simulink model "PubIfDecisionTOS_MDL"  (R2020b)
settings: configuration reference "DspaceConfig" (kept outside this file)
PostLoadFcn:
  | if any(exist('dsrtsu_mdlpostloadfcn', 'file') ~= 0), dsrtsu_mdlpostloadfcn('Execute', bdroot); end
InitFcn:
  | , if any(exist('dsmpb_private', 'file') ~= 0), dsmpb_private('dsmpb_mdlclblib', 'Init', bdroot); end,
undefined symbols (not defined in the file or in its folder): C_TOS_ACCEgoRAxletoFbumplength_m, C_TOS_ACCTargetFront_Flag, C_TOS_AEBJAPedObjDxThre_Val, C_TOS_AEBJAPedObjDyThre_Val, C_TOS_AEBJATargetSize_Val, C_TOS_AEBJAVehObjDxThre_Val, C_TOS_AEBJAVehObjDyThre_Val, C_TOS_AEBJuncPedTargetSize_Val, C_TOS_AEBLatObjDxThre_Val, C_TOS_AEBLatPedDyThre_Val, C_TOS_AEBLatTargetSize_Val, C_TOS_AEBLongTargetInEgoFront_Flag, C_TOS_axAbsGround_Parameter, C_TOS_CameraConfirmedFlag, C_TOS_CNsubjWidth, C_TOS_CurrentLaneCoreMinWidth_Val, C_TOS_CutInProb_Val_Zero, C_TOS_CutOutProb_Val_Zero, C_TOS_D2R_Val, C_TOS_DefaultValueObjectToCenterLine_dy, C_TOS_EgoCarWidth_Val, C_TOS_EgoDxRefPoint_m, C_TOS_EgoRAxletoFbumplength_m, C_TOS_HalfWidthVehicle_Con, C_TOS_HWA_CurrentLaneFlag, C_TOS_HWA_LeftLaneFlag, C_TOS_HWA_MovingDir_Vaild, C_TOS_HWA_MovState_Vaild, C_TOS_HWA_RightLaneFlag, C_TOS_LaneLineCourseErrorFront, C_TOS_LaneLineCourseErrorRear, C_TOS_MotorbikeDefaultWidth_m, C_TOS_NumberOfEffectiveTargets, C_TOS_Obj_Age_Val, C_TOS_Objdx_Constraint_Val, C_TOS_ObjectDefaultWidth_m, C_TOS_ObjInCurrentLane_Val, C_TOS_ObjInCurrentLaneValid, C_TOS_ObjInLeftLaneValid, C_TOS_ObjInRightLaneValid, C_TOS_ObjNotInCurrentLane_Val, C_TOS_ObjNotREElementType, C_TOS_ObjPredictDis_dy_ConstantVal_Zeros, C_TOS_ObjToCenterLine_ConstantVal_Zeros, C_TOS_OFMObjIDInvilad_Val, C_TOS_PIL_LatDisCons_Val_zero, C_TOS_PIL_ObjectCutInFlag_b, C_TOS_PIL_ObjectCutOutFlag_b, C_TOS_PIL_ObjLaneProb_al_Val, C_TOS_PP_ObjFusType_FC_Confirm_b, C_TOS_PP_ObjFusType_FC_FR_Confirm_b, C_TOS_PP_ObjFusType_FR_Confirm_b, C_TOS_RE_80BoolDefault_Val, C_TOS_RE_80Single181Default_Val, C_TOS_RE_80Single255Default_Val, C_TOS_RE_80Uint8Default_Val, C_TOS_RE_D2R, C_TOS_RE_D_180_Val, C_TOS_RE_InvalidObjectID_Val, C_TOS_RE_InvalidTargetChainDir_Val ... (+142)
libraries: simulink x1650, TOS_LIB x361, canfdmsglib x14
(part 56 of 69)

== system PubIfDecisionTOS_MDL/TOS_20201112/TOS_2012080320/TOS/LC_LCKie_ELK/TOS_HWA/LeftLane/TOS_HWA_LeftLane/TOS_HWA_LeftLane/TOS_HWA/HWA_LeftLane/HWA_LeftLane_Rear ==
  HWA_MovState_InternalSig : Inport
  Object_Fus_Type : Inport  Port=2
  TOS_TLJ_LeftLaneConfirm_Flag : Inport  Port=3
  HWA_MovingDir_InternalSig : Inport  Port=4
  Object_DY : Inport  Port=5
  Object_DX : Inport  Port=6
  HWA_InLeftLane_Flag : Subsystem
  HWA_LeftFront_Default : Subsystem
  HWA_LeftRear_DyConfirm : Subsystem
  HWA_LeftRear_FusionType : Subsystem
  HWA_LeftRear_MovState : Subsystem
  HWA_LeftRear_TargetMovingDir : Subsystem
  Logical Operator4 : Logic  Inputs=5  AllPortsSameDT=off  OutDataTypeStr=boolean
  Object_DX1 : InportShadow  Port=6
  TOS_HWA_LeftFront_TargConfirm_b : Outport
  TOS_HWA_LeftFront_FusType_ObserVale : Outport  Port=2
  TOS_HWA_InLeftLane_Front_Flag_ObserVale : Outport  Port=3
  TOS_HWA_LeftFront_TargMovDir_ObserVale : Outport  Port=4
  TOS_HWA_LeftRear_TargConfirm_b : Outport  Port=5
  TOS_HWA_LeftRear_MovState_ObserVale : Outport  Port=6
  TOS_HWA_LeftRear_FusionType_ObserVale : Outport  Port=7
  TOS_HWA_InLeftLane_Rear_Flag_ObserVale : Outport  Port=8
  TOS_HWA_LeftRear_TargetMovingDir_ObserVale : Outport  Port=9
  TOS_HWA_LeftRear_DyConfirm_ObserVale : Outport  Port=10
  wires:
  Object_DX1/1 -> HWA_LeftRear_FusionType/2(Object_DX)
  Object_DX/1 -> HWA_LeftRear_DyConfirm/2(Object_DX)
  HWA_LeftRear_DyConfirm/1(TOS_HWA_LeftRear_DyConfirm) -> Logical Operator4/5, [TOS_HWA_LeftRear_DyConfirm_ObserVale]
  HWA_LeftRear_TargetMovingDir/1(TOS_HWA_LeftRear_TargetMovingDir) -> Logical Operator4/4, [TOS_HWA_LeftRear_TargetMovingDir_ObserVale]
  HWA_InLeftLane_Flag/1(TOS_HWA_InLeftLane_Flag) -> Logical Operator4/3, [TOS_HWA_InLeftLane_Flag_ObserVale]
  HWA_LeftRear_FusionType/1(TOS_HWA_LeftRear_FusionType) -> Logical Operator4/2, [TOS_HWA_LeftRear_FusionType_ObserVale]
  HWA_LeftRear_MovState/1(TOS_HWA_LeftRear_MovState) -> Logical Operator4/1, [TOS_HWA_LeftRear_MovState_ObserVale]
  Object_DY/1 -> HWA_LeftRear_DyConfirm/1(Object_DY)
  HWA_MovingDir_InternalSig/1 -> HWA_LeftRear_TargetMovingDir/1(HWA_MovingDir_InternalSig)
  TOS_TLJ_LeftLaneConfirm_Flag/1 -> HWA_InLeftLane_Flag/1(HWA_InRightLane)
  Object_Fus_Type/1 -> HWA_LeftRear_FusionType/1(Object_FusType)
  HWA_MovState_InternalSig/1 -> HWA_LeftRear_MovState/1(HWA_MovState_InternalSig)
  [TOS_HWA_LeftRear_DyConfirm_ObserVale] -> TOS_HWA_LeftRear_DyConfirm_ObserVale/1  "TOS_HWA_LeftRear_DyConfirm_ObserVale"
  [TOS_HWA_LeftRear_TargetMovingDir_ObserVale] -> TOS_HWA_LeftRear_TargetMovingDir_ObserVale/1  "TOS_HWA_LeftRear_TargetMovingDir_ObserVale"
  Logical Operator4/1 -> TOS_HWA_LeftRear_TargConfirm_b/1  "TOS_HWA_LeftRear_TargConfirm_b"
  HWA_LeftFront_Default/3(TOS_HWA_InLeftLane_Front_Flag_ObserVale) -> TOS_HWA_InLeftLane_Front_Flag_ObserVale/1  "TOS_HWA_InLeftLane_Front_Flag_ObserVale"
  HWA_LeftFront_Default/2(TOS_HWA_LeftFront_FusType_ObserVale) -> TOS_HWA_LeftFront_FusType_ObserVale/1  "TOS_HWA_LeftFront_FusType_ObserVale"
  [TOS_HWA_InLeftLane_Flag_ObserVale] -> TOS_HWA_InLeftLane_Rear_Flag_ObserVale/1  "TOS_HWA_InLeftLane_Rear_Flag_ObserVale"
  HWA_LeftFront_Default/1(TOS_HWA_LeftFront_TargConfirm_b) -> TOS_HWA_LeftFront_TargConfirm_b/1  "TOS_HWA_LeftFront_TargConfirm_b"
  HWA_LeftFront_Default/4(TOS_HWA_LeftFront_TargMovDir_ObserVale) -> TOS_HWA_LeftFront_TargMovDir_ObserVale/1  "TOS_HWA_LeftFront_TargMovDir_ObserVale"
  [TOS_HWA_LeftRear_MovState_ObserVale] -> TOS_HWA_LeftRear_MovState_ObserVale/1  "TOS_HWA_LeftRear_MovState_ObserVale"
  [TOS_HWA_LeftRear_FusionType_ObserVale] -> TOS_HWA_LeftRear_FusionType_ObserVale/1  "TOS_HWA_LeftRear_FusionType_ObserVale"

== system PubIfDecisionTOS_MDL/TOS_20201112/TOS_2012080320/TOS/LC_LCKie_ELK/TOS_HWA/LeftLane/TOS_HWA_LeftLane/TOS_HWA_LeftLane/TOS_HWA/HWA_LeftLane/HWA_MovState ==
  note: Fun：计算目标相对于大地的绝对速度
      |
      | fun1:目标绝对速度 = 目标相对速度（融合输出）+ 自车速度
      |
      | （目标相对速度 = 目标速度 - 自车速度）
  Object_VX : Inport
  Object_VY : Inport  Port=2
  VIE_EgoVelocity : Inport  Port=3
  Add : Sum
  Compare To Constant1 : simulink/Logic and Bit Operations/Compare To Constant  relop=>  const=1.5  OutDataTypeStr=boolean
      settings: AttributesFormatString== 1.5
  Terminator : Terminator
  HWA_MovState_InternalSig : Outport
  wires:
  Compare To Constant1/1 -> HWA_MovState_InternalSig/1
  Object_VY/1 -> Terminator/1
  Add/1 -> Compare To Constant1/1
  VIE_EgoVelocity/1 -> Add/2
  Object_VX/1 -> Add/1

== system PubIfDecisionTOS_MDL/TOS_20201112/TOS_2012080320/TOS/LC_LCKie_ELK/TOS_HWA/LeftLane/TOS_HWA_LeftLane/TOS_HWA_LeftLane/TOS_HWA/HWA_LeftLane/HWA_MovingDir ==
  note: OncomingDir
  note: SameDir
  object_MovingState : Inport
  PP_ObjMovingDirSignalProcessing : Inport  Port=2
  Object_HeadingAngle : Inport  Port=3
  Object_VX : Inport  Port=4
  Object_VY : Inport  Port=5
  VIE_EgoVelocity : Inport  Port=6
  Abs{,1..3} (4 alike) : Abs
  Add : Sum
  Add1 : Sum
  Compare To Constant : simulink/Logic and Bit Operations/Compare To Constant  relop===  const=ObjectMovingOrientation_E.SameDir  OutDataTypeStr=boolean
      settings: AttributesFormatString=ObjectMovingOrientation_E.SameDir = 1
  Compare To Constant1 : simulink/Logic and Bit Operations/Compare To Constant  relop===  const=OFM_OBJ_MOVINGSTATE_E.MOVING  OutDataTypeStr=boolean
      settings: AttributesFormatString=OFM_OBJ_MOVINGSTATE_E.MOVING = 2
  Compare To Constant2 : simulink/Logic and Bit Operations/Compare To Constant  relop=>=  const=P_TOS_ObjInSameDirYawAngMinThre_Val  OutDataTypeStr=boolean
      settings: AttributesFormatString=P_TOS_ObjInSameDirYawAngMinThre_Val = 0
  Compare To Constant3 : simulink/Logic and Bit Operations/Compare To Constant  relop=<=  const=P_TOS_ObjInSameDirYawAngMaxThre_Val  OutDataTypeStr=boolean
      settings: AttributesFormatString=P_TOS_ObjInSameDirYawAngMaxThre_Val = 45
  Compare To Constant4 : simulink/Logic and Bit Operations/Compare To Constant  relop===  const=OFM_OBJ_MOVINGSTATE_E.MOVING_SLOWLY  OutDataTypeStr=boolean
      settings: AttributesFormatString=OFM_OBJ_MOVINGSTATE_E.MOVING_SLOWLY = 5
  Compare To Constant5 : simulink/Logic and Bit Operations/Compare To Constant  relop===  const=ObjectMovingOrientation_E.OnComingDir  OutDataTypeStr=boolean
      settings: AttributesFormatString=ObjectMovingOrientation_E.OnComingDir = 2
  Compare To Constant6 : simulink/Logic and Bit Operations/Compare To Constant  relop=>=  const=P_TOS_ObjLatCroYawAngMaxThre_Val  OutDataTypeStr=boolean
      settings: AttributesFormatString=P_TOS_ObjLatCroYawAngMaxThre_Val = 135
  Compare To Constant7 : simulink/Logic and Bit Operations/Compare To Constant  relop=<=  const=P_TOS_ObjOncomingYawAngMaxThre_Val  OutDataTypeStr=boolean
      settings: AttributesFormatString=P_TOS_ObjOncomingYawAngMaxThre_Val = 180
  Compare To Constant8 : simulink/Logic and Bit Operations/Compare To Constant  relop=<  const=P_TOS_SameDirVyOffset_Val  OutDataTypeStr=boolean
      settings: AttributesFormatString=P_TOS_SameDirVyOffset_Val = 2
  Constant : Constant  OutDataTypeStr=boolean
  Constant1 : Constant  Value=P_TOS_SameDirVxvOffset_Val
      settings: AttributesFormatString=P_TOS_AEBLong_SameDirVxvOffset_Val = 0.2
  Constant2 : Constant  Value=P_TOS_OncomingDirVxvOffset_Val
      settings: AttributesFormatString=P_TOS_OncomingDirVxvOffset_Val = 0.2
  Data Type Conversion1 : DataTypeConversion  OutDataTypeStr=Enum: ObjectMovingOrientation_E
  Data Type Conversion2 : DataTypeConversion  OutDataTypeStr=Enum: OFM_OBJ_MOVINGSTATE_E
  Logical Operator{,3..4,7} (4 alike) : Logic  AllPortsSameDT=off  OutDataTypeStr=boolean
  Logical Operator1 : Logic  Operator=OR  AllPortsSameDT=off  OutDataTypeStr=boolean
  Logical Operator2 : Logic  Operator=OR  AllPortsSameDT=off  OutDataTypeStr=boolean
  Logical Operator5 : Logic  Operator=OR  AllPortsSameDT=off  OutDataTypeStr=boolean
  Logical Operator6 : Logic  Operator=OR  Inputs=4  AllPortsSameDT=off  OutDataTypeStr=boolean
  Relational Operator : RelationalOperator  Operator=<  OutDataTypeStr=boolean  RndMeth=Simplest
  Relational Operator1 : RelationalOperator  Operator=>  OutDataTypeStr=boolean  RndMeth=Simplest
  Switch : Switch  Criteria=u2 > Threshold
  HWA_MovingDir_InternalSig : Outport
  wires:
  Abs3/1 -> Add1/1
  [VIE_EgoVelocity] -> Relational Operator1/2
  Add1/1 -> Relational Operator1/1
  Logical Operator7/1 -> Logical Operator6/4
  Relational Operator1/1 -> Logical Operator7/2
  Logical Operator/1 -> Logical Operator6/3
  [Object_VX] -> Abs3/1
  Abs2/1 -> Compare To Constant8/1
  Object_VY/1 -> Abs2/1
  Add/1 -> Relational Operator/1
  Constant1/1 -> Add/2
  Object_VX/1 -> Abs1/1, [Object_VX]
  VIE_EgoVelocity/1 -> [VIE_EgoVelocity], Relational Operator/2
  Abs1/1 -> Add/1
  Compare To Constant8/1 -> Logical Operator/2, Logical Operator7/1
  Relational Operator/1 -> Logical Operator/1
  Constant2/1 -> Add1/2
  Logical Operator1/1 -> Logical Operator6/2
  Logical Operator5/1 -> Logical Operator6/1
  Compare To Constant5/1 -> Logical Operator5/1
  Logical Operator4/1 -> Logical Operator5/2
  Compare To Constant7/1 -> Logical Operator4/2
  Compare To Constant6/1 -> Logical Operator4/1
  PP_ObjMovingDirSignalProcessing/1 -> Data Type Conversion1/1
  Logical Operator6/1 -> Switch/1
  Data Type Conversion1/1 -> Compare To Constant5/1, Compare To Constant/1
  Compare To Constant2/1 -> Logical Operator3/1
  Compare To Constant3/1 -> Logical Operator3/2
  Abs/1 -> Compare To Constant6/1, Compare To Constant3/1, Compare To Constant2/1, Compare To Constant7/1
  Object_HeadingAngle/1 -> Abs/1
  Compare To Constant/1 -> Logical Operator1/1
  Logical Operator3/1 -> Logical Operator1/2
  Data Type Conversion2/1 -> Compare To Constant4/1, Compare To Constant1/1
  object_MovingState/1 -> Data Type Conversion2/1
  Compare To Constant4/1 -> Logical Operator2/2
  Compare To Constant1/1 -> Logical Operator2/1
  Logical Operator2/1 -> Switch/2
  Switch/1 -> HWA_MovingDir_InternalSig/1
  Constant/1 -> Switch/3

== system PubIfDecisionTOS_MDL/TOS_20201112/TOS_2012080320/TOS/LC_LCKie_ELK/TOS_HWA/RightLane/TOS_HWA_RightLane/TOS_HWA_RightLane/TOS_HWA/HWA_RightLane/HWA_MovState ==
  note: Fun：计算目标相对于大地的绝对速度
      |
      | fun1:目标绝对速度 = 目标相对速度（融合输出）+ 自车速度
      |
      | （目标相对速度 = 目标速度 - 自车速度）
  Object_VX : Inport
  Object_VY : Inport  Port=2
  VIE_EgoVelocity : Inport  Port=3
  Add : Sum
  Compare To Constant1 : simulink/Logic and Bit Operations/Compare To Constant  relop=>  const=1.5  OutDataTypeStr=boolean
      settings: AttributesFormatString== 1.5
  Terminator : Terminator
  HWA_MovState_InternalSig : Outport
  wires:
  Object_VX/1 -> Add/1
  VIE_EgoVelocity/1 -> Add/2
  Add/1 -> Compare To Constant1/1
  Object_VY/1 -> Terminator/1
  Compare To Constant1/1 -> HWA_MovState_InternalSig/1

== system PubIfDecisionTOS_MDL/TOS_20201112/TOS_2012080320/TOS/LC_LCKie_ELK/TOS_HWA/RightLane/TOS_HWA_RightLane/TOS_HWA_RightLane/TOS_HWA/HWA_RightLane/HWA_MovingDir ==
  note: SameDir
  note: OncomingDir
  object_MovingState : Inport
  PP_ObjMovingDirSignalProcessing : Inport  Port=2
  Object_HeadingAngle : Inport  Port=3
  Object_VX : Inport  Port=4
  Object_VY : Inport  Port=5
  VIE_EgoVelocity : Inport  Port=6
  Abs{,1..3} (4 alike) : Abs
  Add : Sum
  Add1 : Sum
  Compare To Constant : simulink/Logic and Bit Operations/Compare To Constant  relop===  const=ObjectMovingOrientation_E.SameDir  OutDataTypeStr=boolean
      settings: AttributesFormatString=ObjectMovingOrientation_E.SameDir = 1
  Compare To Constant1 : simulink/Logic and Bit Operations/Compare To Constant  relop===  const=OFM_OBJ_MOVINGSTATE_E.MOVING  OutDataTypeStr=boolean
      settings: AttributesFormatString=OFM_OBJ_MOVINGSTATE_E.MOVING = 2
  Compare To Constant2 : simulink/Logic and Bit Operations/Compare To Constant  relop=>=  const=P_TOS_ObjInSameDirYawAngMinThre_Val  OutDataTypeStr=boolean
      settings: AttributesFormatString=P_TOS_ObjInSameDirYawAngMinThre_Val = 0
  Compare To Constant3 : simulink/Logic and Bit Operations/Compare To Constant  relop=<=  const=P_TOS_ObjInSameDirYawAngMaxThre_Val  OutDataTypeStr=boolean
      settings: AttributesFormatString=P_TOS_ObjInSameDirYawAngMaxThre_Val = 45
  Compare To Constant4 : simulink/Logic and Bit Operations/Compare To Constant  relop===  const=OFM_OBJ_MOVINGSTATE_E.MOVING_SLOWLY  OutDataTypeStr=boolean
      settings: AttributesFormatString=OFM_OBJ_MOVINGSTATE_E.MOVING_SLOWLY = 5
  Compare To Constant5 : simulink/Logic and Bit Operations/Compare To Constant  relop===  const=ObjectMovingOrientation_E.OnComingDir  OutDataTypeStr=boolean
      settings: AttributesFormatString=ObjectMovingOrientation_E.OnComingDir = 2
  Compare To Constant6 : simulink/Logic and Bit Operations/Compare To Constant  relop=>=  const=P_TOS_ObjLatCroYawAngMaxThre_Val  OutDataTypeStr=boolean
      settings: AttributesFormatString=P_TOS_ObjLatCroYawAngMaxThre_Val = 135
  Compare To Constant7 : simulink/Logic and Bit Operations/Compare To Constant  relop=<=  const=P_TOS_ObjOncomingYawAngMaxThre_Val  OutDataTypeStr=boolean
      settings: AttributesFormatString=P_TOS_ObjOncomingYawAngMaxThre_Val = 180
  Compare To Constant8 : simulink/Logic and Bit Operations/Compare To Constant  relop=<  const=P_TOS_SameDirVyOffset_Val  OutDataTypeStr=boolean
      settings: AttributesFormatString=P_TOS_SameDirVyOffset_Val = 2
  Constant : Constant  OutDataTypeStr=boolean
  Constant1 : Constant  Value=P_TOS_SameDirVxvOffset_Val
      settings: AttributesFormatString=P_TOS_AEBLong_SameDirVxvOffset_Val = 0.2
  Constant2 : Constant  Value=P_TOS_OncomingDirVxvOffset_Val
      settings: AttributesFormatString=P_TOS_OncomingDirVxvOffset_Val = 0.2
  Data Type Conversion1 : DataTypeConversion  OutDataTypeStr=Enum: ObjectMovingOrientation_E
  Data Type Conversion2 : DataTypeConversion  OutDataTypeStr=Enum: OFM_OBJ_MOVINGSTATE_E
  Logical Operator{,3..4,7} (4 alike) : Logic  AllPortsSameDT=off  OutDataTypeStr=boolean
  Logical Operator1 : Logic  Operator=OR  AllPortsSameDT=off  OutDataTypeStr=boolean
  Logical Operator2 : Logic  Operator=OR  AllPortsSameDT=off  OutDataTypeStr=boolean
  Logical Operator5 : Logic  Operator=OR  AllPortsSameDT=off  OutDataTypeStr=boolean
  Logical Operator6 : Logic  Operator=OR  Inputs=4  AllPortsSameDT=off  OutDataTypeStr=boolean
  Relational Operator : RelationalOperator  Operator=<  OutDataTypeStr=boolean  RndMeth=Simplest
  Relational Operator1 : RelationalOperator  Operator=>  OutDataTypeStr=boolean  RndMeth=Simplest
  Switch : Switch  Criteria=u2 > Threshold
  HWA_MovingDir_InternalSig : Outport
  wires:
  Constant/1 -> Switch/3
  Switch/1 -> HWA_MovingDir_InternalSig/1
  Logical Operator2/1 -> Switch/2
  Compare To Constant1/1 -> Logical Operator2/1
  Compare To Constant4/1 -> Logical Operator2/2
  object_MovingState/1 -> Data Type Conversion2/1
  Data Type Conversion2/1 -> Compare To Constant1/1, Compare To Constant4/1
  Logical Operator3/1 -> Logical Operator1/2
  Compare To Constant/1 -> Logical Operator1/1
  Object_HeadingAngle/1 -> Abs/1
  Abs/1 -> Compare To Constant7/1, Compare To Constant2/1, Compare To Constant3/1, Compare To Constant6/1
  Compare To Constant3/1 -> Logical Operator3/2
  Compare To Constant2/1 -> Logical Operator3/1
  Data Type Conversion1/1 -> Compare To Constant/1, Compare To Constant5/1
  Logical Operator6/1 -> Switch/1
  PP_ObjMovingDirSignalProcessing/1 -> Data Type Conversion1/1
  Compare To Constant6/1 -> Logical Operator4/1
  Compare To Constant7/1 -> Logical Operator4/2
  Logical Operator4/1 -> Logical Operator5/2
  Compare To Constant5/1 -> Logical Operator5/1
  Logical Operator5/1 -> Logical Operator6/1
  Logical Operator1/1 -> Logical Operator6/2
  Constant2/1 -> Add1/2
  Relational Operator/1 -> Logical Operator/1
  Compare To Constant8/1 -> Logical Operator7/1, Logical Operator/2
  Abs1/1 -> Add/1
  VIE_EgoVelocity/1 -> Relational Operator/2, [VIE_EgoVelocity]
  Object_VX/1 -> [Object_VX], Abs1/1
  Constant1/1 -> Add/2
  Add/1 -> Relational Operator/1
  Object_VY/1 -> Abs2/1
  Abs2/1 -> Compare To Constant8/1
  [Object_VX] -> Abs3/1
  Logical Operator/1 -> Logical Operator6/3
  Relational Operator1/1 -> Logical Operator7/2
  Logical Operator7/1 -> Logical Operator6/4
  Add1/1 -> Relational Operator1/1
  [VIE_EgoVelocity] -> Relational Operator1/2
  Abs3/1 -> Add1/1

== system PubIfDecisionTOS_MDL/TOS_20201112/TOS_2012080320/TOS/LC_LCKie_ELK/TOS_HWA/RightLane/TOS_HWA_RightLane/TOS_HWA_RightLane/TOS_HWA/HWA_RightLane/HWA_RightLane_Default ==
  Constant{,1..9} (10 alike) : Constant  Value=0  OutDataTypeStr=boolean
  TOS_HWA_RightFront_TargConfirm_b : Outport
  TOS_HWA_RightFront_FusType_ObserVale : Outport  Port=2
  TOS_HWA_InRightLane_Front_Flag_ObserVale : Outport  Port=3
  TOS_HWA_RightFront_TargMovDir_ObserVale : Outport  Port=4
  TOS_HWA_RightRear_TargConfirm_b : Outport  Port=5
  TOS_HWA_RightRear_MovState_ObserVale : Outport  Port=6
  TOS_HWA_RightRear_FusionType_ObserVale : Outport  Port=7
  TOS_HWA_InRightLane_Rear_Flag_ObserVale : Outport  Port=8
  TOS_HWA_RightRear_TargetMovingDir_ObserVale : Outport  Port=9
  TOS_HWA_RightRear_DyConfirm_ObserVale : Outport  Port=10
  wires:
  Constant3/1 -> TOS_HWA_RightFront_TargMovDir_ObserVale/1  "TOS_HWA_RightFront_TargMovDir_ObserVale"
  Constant/1 -> TOS_HWA_RightFront_TargConfirm_b/1  "TOS_HWA_RightFront_TargConfirm_b"
  Constant1/1 -> TOS_HWA_RightFront_FusType_ObserVale/1  "TOS_HWA_RightFront_FusType_ObserVale"
  Constant6/1 -> TOS_HWA_RightRear_FusionType_ObserVale/1  "TOS_HWA_RightRear_FusionType_ObserVale"
  Constant7/1 -> TOS_HWA_InRightLane_Rear_Flag_ObserVale/1  "TOS_HWA_InRightLane_Rear_Flag_ObserVale"
  Constant9/1 -> TOS_HWA_RightRear_DyConfirm_ObserVale/1  "TOS_HWA_RightRear_DyConfirm_ObserVale"
  Constant8/1 -> TOS_HWA_RightRear_TargetMovingDir_ObserVale/1  "TOS_HWA_RightRear_TargetMovingDir_ObserVale"
  Constant5/1 -> TOS_HWA_RightRear_MovState_ObserVale/1  "TOS_HWA_RightRear_MovState_ObserVale"
  Constant2/1 -> TOS_HWA_InRightLane_Front_Flag_ObserVale/1  "TOS_HWA_InRightLane_Front_Flag_ObserVale"
  Constant4/1 -> TOS_HWA_RightRear_TargConfirm_b/1  "TOS_HWA_RightRear_TargConfirm_b"

== system PubIfDecisionTOS_MDL/TOS_20201112/TOS_2012080320/TOS/LC_LCKie_ELK/TOS_HWA/RightLane/TOS_HWA_RightLane/TOS_HWA_RightLane/TOS_HWA/HWA_RightLane/HWA_RightLane_Front ==
  object_MovingState : Inport
  PP_ObjFusType_FR_Confirm : Inport  Port=2
  PP_ObjFusType_FC_Confirm : Inport  Port=3
  HWA_MovState_InternalSig : Inport  Port=4
  TOS_TLJ_RightLaneConfirm_Flag : Inport  Port=5
  HWA_MovingDir_InternalSig : Inport  Port=6
  Object_DX : Inport  Port=7
  Bus Creator : BusCreator  Inputs=7
  Bus Selector : BusSelector  OutputSignals=object_MovingState,PP_ObjFusType_FR_Confirm,PP_ObjFusType_FC_Confirm,HWA_MovState_InternalSig,Object_DX
  Bus Selector1 : BusSelector  OutputSignals=TOS_TLJ_RightLaneConfirm_Flag
  Bus Selector2 : BusSelector  OutputSignals=HWA_MovingDir_InternalSig
  HWA_InRightLane_Flag : Subsystem
  HWA_RightFront_FusType : Subsystem
  HWA_RightFront_TargMovDir : Subsystem
  HWA_RightRear_Default : Subsystem
  Logical Operator4 : Logic  Inputs=3  AllPortsSameDT=off  OutDataTypeStr=boolean
  TOS_HWA_RightFront_TargConfirm_b : Outport
  TOS_HWA_RightFront_FusType_ObserVale : Outport  Port=2
  TOS_HWA_InRightLane_Front_Flag_ObserVale : Outport  Port=3
  TOS_HWA_RightFront_TargMovDir_ObserVale : Outport  Port=4
  TOS_HWA_RightRear_TargConfirm_b : Outport  Port=5
  TOS_HWA_RightRear_MovState_ObserVale : Outport  Port=6
  TOS_HWA_RightRear_FusionType_ObserVale : Outport  Port=7
  TOS_HWA_InRightLane_Rear_Flag_ObserVale : Outport  Port=8
  TOS_HWA_RightRear_TargetMovingDir_ObserVale : Outport  Port=9
  TOS_HWA_RightRear_DyConfirm_ObserVale : Outport  Port=10
  wires:
  object_MovingState/1 -> Bus Creator/1  "object_MovingState"
  HWA_MovingDir_InternalSig/1 -> Bus Creator/6  "HWA_MovingDir_InternalSig"
  TOS_TLJ_RightLaneConfirm_Flag/1 -> Bus Creator/5  "TOS_TLJ_RightLaneConfirm_Flag"
  HWA_MovState_InternalSig/1 -> Bus Creator/4  "HWA_MovState_InternalSig"
  PP_ObjFusType_FC_Confirm/1 -> Bus Creator/3  "PP_ObjFusType_FC_Confirm"
  PP_ObjFusType_FR_Confirm/1 -> Bus Creator/2  "PP_ObjFusType_FR_Confirm"
  Bus Creator/1 -> Bus Selector2/1, Bus Selector1/1, Bus Selector/1
  Bus Selector/1 -> HWA_RightFront_FusType/1(object_MovingState)  "<object_MovingState>"
  Bus Selector/2 -> HWA_RightFront_FusType/2(PP_ObjFusType_FR_Confirm)  "<PP_ObjFusType_FR_Confirm>"
  Bus Selector/3 -> HWA_RightFront_FusType/3(PP_ObjFusType_FC_Confirm)  "<PP_ObjFusType_FC_Confirm>"
  Bus Selector/4 -> HWA_RightFront_FusType/4(HWA_MovState_InternalSig)  "<HWA_MovState_InternalSig>"
  Bus Selector1/1 -> HWA_InRightLane_Flag/1(TOS_TLJ_RightLaneConfirm_Flag)  "<TOS_TLJ_RightLaneConfirm_Flag>"
  Bus Selector2/1 -> HWA_RightFront_TargMovDir/1(HWA_MovingDir_InternalSig)  "<HWA_MovingDir_InternalSig>"
  HWA_RightFront_FusType/1(TOS_HWA_RightFront_FusType) -> [TOS_HWA_RightFront_FusType_ObserVale], Logical Operator4/1
  HWA_InRightLane_Flag/1(TOS_HWA_InRightLane_Flag) -> [TOS_HWA_InRightLane_Flag_ObserVale], Logical Operator4/2
  HWA_RightFront_TargMovDir/1(TOS_HWA_RightFront_TargMovDir) -> [TOS_HWA_RightFront_TargMovDir_ObserVale], Logical Operator4/3
  Logical Operator4/1 -> TOS_HWA_RightFront_TargConfirm_b/1  "TOS_HWA_RightFront_TargConfirm_b"
  [TOS_HWA_RightFront_FusType_ObserVale] -> TOS_HWA_RightFront_FusType_ObserVale/1  "TOS_HWA_RightFront_FusType_ObserVale"
  [TOS_HWA_InRightLane_Flag_ObserVale] -> TOS_HWA_InRightLane_Front_Flag_ObserVale/1  "TOS_HWA_InRightLane_Front_Flag_ObserVale"
  [TOS_HWA_RightFront_TargMovDir_ObserVale] -> TOS_HWA_RightFront_TargMovDir_ObserVale/1  "TOS_HWA_RightFront_TargMovDir_ObserVale"
  HWA_RightRear_Default/1(TOS_HWA_RightRear_TargConfirm_b) -> TOS_HWA_RightRear_TargConfirm_b/1  "TOS_HWA_RightRear_TargConfirm_b"
  HWA_RightRear_Default/2(TOS_HWA_RightRear_MovState_ObserVale) -> TOS_HWA_RightRear_MovState_ObserVale/1  "TOS_HWA_RightRear_MovState_ObserVale"
  HWA_RightRear_Default/3(TOS_HWA_RightRear_FusionType_ObserVale) -> TOS_HWA_RightRear_FusionType_ObserVale/1  "TOS_HWA_RightRear_FusionType_ObserVale"
  HWA_RightRear_Default/4(TOS_HWA_InRightLane_Rear_Flag_ObserVale) -> TOS_HWA_InRightLane_Rear_Flag_ObserVale/1  "TOS_HWA_InRightLane_Rear_Flag_ObserVale"
  HWA_RightRear_Default/5(TOS_HWA_RightRear_TargetMovingDir_ObserVale) -> TOS_HWA_RightRear_TargetMovingDir_ObserVale/1  "TOS_HWA_RightRear_TargetMovingDir_ObserVale"
  HWA_RightRear_Default/6(TOS_HWA_RightRear_DyConfirm_ObserVale) -> TOS_HWA_RightRear_DyConfirm_ObserVale/1  "TOS_HWA_RightRear_DyConfirm_ObserVale"
  Object_DX/1 -> Bus Creator/7  "Object_DX"
  Bus Selector/5 -> HWA_RightFront_FusType/5(Object_DX)  "<Object_DX>"

== system PubIfDecisionTOS_MDL/TOS_20201112/TOS_2012080320/TOS/LC_LCKie_ELK/TOS_HWA/RightLane/TOS_HWA_RightLane/TOS_HWA_RightLane/TOS_HWA/HWA_RightLane/HWA_RightLane_Rear ==
  HWA_MovState_InternalSig : Inport
  Object_Fus_Type : Inport  Port=2
  TOS_TLJ_RightLaneConfirm_Flag : Inport  Port=3
  HWA_MovingDir_InternalSig : Inport  Port=4
  Object_DY : Inport  Port=5
  Object_DX : Inport  Port=6
  HWA_InRightLane_Flag : Subsystem
  HWA_RightFront_Default : Subsystem
  HWA_RightRear_DyConfirm : Subsystem
  HWA_RightRear_FusionType : Subsystem
  HWA_RightRear_MovState : Subsystem
  HWA_RightRear_TargetMovingDir : Subsystem
  Logical Operator4 : Logic  Inputs=5  AllPortsSameDT=off  OutDataTypeStr=boolean
  Object_DX1 : InportShadow  Port=6
  TOS_HWA_RightFront_TargConfirm_b : Outport
  TOS_HWA_RightFront_FusType_ObserVale : Outport  Port=2
  TOS_HWA_InRightLane_Front_Flag_ObserVale : Outport  Port=3
  TOS_HWA_RightFront_TargMovDir_ObserVale : Outport  Port=4
  TOS_HWA_RightRear_TargConfirm_b : Outport  Port=5
  TOS_HWA_RightRear_MovState_ObserVale : Outport  Port=6
  TOS_HWA_RightRear_FusionType_ObserVale : Outport  Port=7
  TOS_HWA_InRightLane_Rear_Flag_ObserVale : Outport  Port=8
  TOS_HWA_RightRear_TargetMovingDir_ObserVale : Outport  Port=9
  TOS_HWA_RightRear_DyConfirm_ObserVale : Outport  Port=10
  wires:
  HWA_MovState_InternalSig/1 -> HWA_RightRear_MovState/1(HWA_MovState_InternalSig)
  Object_Fus_Type/1 -> HWA_RightRear_FusionType/1(Object_FusType)
  TOS_TLJ_RightLaneConfirm_Flag/1 -> HWA_InRightLane_Flag/1(TOS_TLJ_RightLaneConfirm_Flag)
  HWA_MovingDir_InternalSig/1 -> HWA_RightRear_TargetMovingDir/1(HWA_MovingDir_InternalSig)
  Object_DY/1 -> HWA_RightRear_DyConfirm/1(Object_DY)
  [TOS_HWA_RightRear_MovState_ObserVale] -> TOS_HWA_RightRear_MovState_ObserVale/1  "TOS_HWA_RightRear_MovState_ObserVale"
  [TOS_HWA_RightRear_FusionType_ObserVale] -> TOS_HWA_RightRear_FusionType_ObserVale/1  "TOS_HWA_RightRear_FusionType_ObserVale"
  [TOS_HWA_InRightLane_Flag_ObserVale] -> TOS_HWA_InRightLane_Rear_Flag_ObserVale/1  "TOS_HWA_InRightLane_Rear_Flag_ObserVale"
  HWA_RightRear_MovState/1(TOS_HWA_RightRear_MovState) -> [TOS_HWA_RightRear_MovState_ObserVale], Logical Operator4/1
  HWA_RightRear_FusionType/1(TOS_HWA_RightRear_FusionType) -> [TOS_HWA_RightRear_FusionType_ObserVale], Logical Operator4/2
  HWA_InRightLane_Flag/1(TOS_HWA_InRightLane_Flag) -> [TOS_HWA_InRightLane_Flag_ObserVale], Logical Operator4/3
  HWA_RightRear_TargetMovingDir/1(TOS_HWA_RightRear_TargetMovingDir) -> [TOS_HWA_RightRear_TargetMovingDir_ObserVale], Logical Operator4/4
  HWA_RightRear_DyConfirm/1(TOS_HWA_RightRear_DyConfirm) -> [TOS_HWA_RightRear_DyConfirm_ObserVale], Logical Operator4/5
  Logical Operator4/1 -> TOS_HWA_RightRear_TargConfirm_b/1  "TOS_HWA_RightRear_TargConfirm_b"
  [TOS_HWA_RightRear_TargetMovingDir_ObserVale] -> TOS_HWA_RightRear_TargetMovingDir_ObserVale/1  "TOS_HWA_RightRear_TargetMovingDir_ObserVale"
  [TOS_HWA_RightRear_DyConfirm_ObserVale] -> TOS_HWA_RightRear_DyConfirm_ObserVale/1  "TOS_HWA_RightRear_DyConfirm_ObserVale"
  Object_DX/1 -> HWA_RightRear_DyConfirm/2(Object_DX)
  HWA_RightFront_Default/1(TOS_HWA_RightFront_TargConfirm_b) -> TOS_HWA_RightFront_TargConfirm_b/1  "TOS_HWA_RightFront_TargConfirm_b"
  HWA_RightFront_Default/2(TOS_HWA_RightFront_FusType_ObserVale) -> TOS_HWA_RightFront_FusType_ObserVale/1  "TOS_HWA_RightFront_FusType_ObserVale"
  HWA_RightFront_Default/3(TOS_HWA_InRightLane_Front_Flag_ObserVale) -> TOS_HWA_InRightLane_Front_Flag_ObserVale/1  "TOS_HWA_InRightLane_Front_Flag_ObserVale"
  HWA_RightFront_Default/4(TOS_HWA_RightFront_TargMovDir_ObserVale) -> TOS_HWA_RightFront_TargMovDir_ObserVale/1  "TOS_HWA_RightFront_TargMovDir_ObserVale"
  Object_DX1/1 -> HWA_RightRear_FusionType/2(Object_DX)

== system PubIfDecisionTOS_MDL/TOS_20201112/TOS_2012080320/TOS/ACC/TOS_ACCCurrentLane/ACC_CurrentLane_Target/TOS_ACC_P0/ACC_P0_Targe/ACC_P0_Targe/TOS_ACC_FusionTypeConfirm/TOS_ACCFusionTypeAborDly/If Action Subsystem ==
  TOS_ACCFusionType : Inport
  Action Port : ActionPort  ActionPortLabel=else
  TOS_ACCFusionTypeFilt : Outport
  wires:
  TOS_ACCFusionType/1 -> TOS_ACCFusionTypeFilt/1

== system PubIfDecisionTOS_MDL/TOS_20201112/TOS_2012080320/TOS/ACC/TOS_ACCCurrentLane/ACC_CurrentLane_Target/TOS_ACC_P0/ACC_P0_Targe/ACC_P0_Targe/TOS_ACC_FusionTypeConfirm/TOS_ACCFusionTypeAborDly/If Action Subsystem1 ==
  TOS_ACCFusionType : Inport
  Action Port : ActionPort  ActionPortLabel=if(u1)
  Constant : Constant  Value=0.15
  Constant4 : Constant  Value=0.05
  StateDelayAbortion : TOS_LIB/StateDelayAbortion  SystemSampleTime=-1  VariantActivationTime=update diagram  Latency=0  AutoFrameSizeCalculation=off
  TOS_ACCFusionTypeFilt : Outport
  wires:
  TOS_ACCFusionType/1 -> StateDelayAbortion/1
  Constant4/1 -> StateDelayAbortion/3
  Constant/1 -> StateDelayAbortion/2
  StateDelayAbortion/1 -> TOS_ACCFusionTypeFilt/1

== system PubIfDecisionTOS_MDL/TOS_20201112/TOS_2012080320/TOS/ACC/TOS_ACCCurrentLane/ACC_CurrentLane_Target/TOS_ACC_P0/ACC_P0_Targe/ACC_P0_Targe/TOS_ACC_ObjTypeConfirm/TOS_ACCObjTypeAborDly/If Action Subsystem ==
  TOS_ACCFusionType : Inport
  Action Port : ActionPort  ActionPortLabel=else
  TOS_ACCFusionTypeFilt : Outport
  wires:
  TOS_ACCFusionType/1 -> TOS_ACCFusionTypeFilt/1

== system PubIfDecisionTOS_MDL/TOS_20201112/TOS_2012080320/TOS/ACC/TOS_ACCCurrentLane/ACC_CurrentLane_Target/TOS_ACC_P0/ACC_P0_Targe/ACC_P0_Targe/TOS_ACC_ObjTypeConfirm/TOS_ACCObjTypeAborDly/If Action Subsystem1 ==
  TOS_ACCFusionType : Inport
  Action Port : ActionPort  ActionPortLabel=if(u1)
  Constant : Constant  Value=0.15
  Constant4 : Constant  Value=0.05
  StateDelayAbortion : TOS_LIB/StateDelayAbortion  SystemSampleTime=-1  VariantActivationTime=update diagram  Latency=0  AutoFrameSizeCalculation=off
  TOS_ACCFusionTypeFilt : Outport
  wires:
  TOS_ACCFusionType/1 -> StateDelayAbortion/1
  Constant4/1 -> StateDelayAbortion/3
  Constant/1 -> StateDelayAbortion/2
  StateDelayAbortion/1 -> TOS_ACCFusionTypeFilt/1

== system PubIfDecisionTOS_MDL/TOS_20201112/TOS_2012080320/TOS/ACC/TOS_ACCCurrentLane/ACC_CurrentLane_Target/TOS_ACC_P0/ACC_P0_Targe/ACC_P0_Targe/TOS_ACC_ObstacleProbConfirm/TOS_ACCObstacleProbAborDly/If Action Subsystem ==
  TOS_ACCFusionType : Inport
  Action Port : ActionPort  ActionPortLabel=else
  TOS_ACCFusionTypeFilt : Outport
  wires:
  TOS_ACCFusionType/1 -> TOS_ACCFusionTypeFilt/1

== system PubIfDecisionTOS_MDL/TOS_20201112/TOS_2012080320/TOS/ACC/TOS_ACCCurrentLane/ACC_CurrentLane_Target/TOS_ACC_P0/ACC_P0_Targe/ACC_P0_Targe/TOS_ACC_ObstacleProbConfirm/TOS_ACCObstacleProbAborDly/If Action Subsystem1 ==
  TOS_ACCFusionType : Inport
  Action Port : ActionPort  ActionPortLabel=if(u1)
  Constant : Constant  Value=0.15
  Constant4 : Constant  Value=0.05
  StateDelayAbortion : TOS_LIB/StateDelayAbortion  SystemSampleTime=-1  VariantActivationTime=update diagram  Latency=0  AutoFrameSizeCalculation=off
  TOS_ACCFusionTypeFilt : Outport
  wires:
  TOS_ACCFusionType/1 -> StateDelayAbortion/1
  Constant4/1 -> StateDelayAbortion/3
  Constant/1 -> StateDelayAbortion/2
  StateDelayAbortion/1 -> TOS_ACCFusionTypeFilt/1

== system PubIfDecisionTOS_MDL/TOS_20201112/TOS_2012080320/TOS/ACC/TOS_ACCCurrentLane/ACC_CurrentLane_Target/TOS_ACC_P0/ACC_P0_Targe/ACC_P0_Targe/TOS_ACC_ObstacleProbConfirm/TOS_ACCObstacleProbAborDly/Subsystem ==
  ACC_TargetP0_ID_K1 : Inport
  ObjectID : Inport  Port=2
  Relational Operator : RelationalOperator  Operator===  OutDataTypeStr=boolean  RndMeth=Simplest
  ACC_SameTargetP0 : Outport
  wires:
  ACC_TargetP0_ID_K1/1 -> Relational Operator/1
  Relational Operator/1 -> ACC_SameTargetP0/1
  ObjectID/1 -> Relational Operator/2

== system PubIfDecisionTOS_MDL/TOS_20201112/TOS_2012080320/TOS/ACC/TOS_ACCCurrentLane/ACC_CurrentLane_Target/TOS_ACC_P0/ACC_P0_Targe/ACC_P0_Targe/TOS_ACC_TargetMovingDirConfirm/TOS_ACCMovingDirAborDly/If Action Subsystem ==
  TOS_ACCMovingDir : Inport
  Action Port : ActionPort  ActionPortLabel=else
  TOS_ACCMovingDirFilt : Outport
  wires:
  TOS_ACCMovingDir/1 -> TOS_ACCMovingDirFilt/1

== system PubIfDecisionTOS_MDL/TOS_20201112/TOS_2012080320/TOS/ACC/TOS_ACCCurrentLane/ACC_CurrentLane_Target/TOS_ACC_P0/ACC_P0_Targe/ACC_P0_Targe/TOS_ACC_TargetMovingDirConfirm/TOS_ACCMovingDirAborDly/If Action Subsystem1 ==
  TOS_ACCMovingDir : Inport
  Action Port : ActionPort  ActionPortLabel=if(u1)
  Constant : Constant  Value=0.15
  Constant4 : Constant  Value=0.05
  StateDelayAbortion : TOS_LIB/StateDelayAbortion  SystemSampleTime=-1  VariantActivationTime=update diagram  Latency=0  AutoFrameSizeCalculation=off
  TOS_ACCMovingDirFilt : Outport
  wires:
  TOS_ACCMovingDir/1 -> StateDelayAbortion/1
  Constant4/1 -> StateDelayAbortion/3
  Constant/1 -> StateDelayAbortion/2
  StateDelayAbortion/1 -> TOS_ACCMovingDirFilt/1

== system PubIfDecisionTOS_MDL/TOS_20201112/TOS_2012080320/TOS/ACC/TOS_ACCCurrentLane/ACC_CurrentLane_Target/TOS_ACC_P0/ACC_P0_Targe/ACC_P0_Targe/TOS_ACC_TargetMovingDirConfirm/TOS_ACCMovingDirAborDly/Subsystem ==
  ACC_TargetP0_ID_K1 : Inport
  ObjectID : Inport  Port=2
  Relational Operator : RelationalOperator  Operator===  OutDataTypeStr=boolean  RndMeth=Simplest
  ACC_SameTargetP0 : Outport
  wires:
  ACC_TargetP0_ID_K1/1 -> Relational Operator/1
  Relational Operator/1 -> ACC_SameTargetP0/1
  ObjectID/1 -> Relational Operator/2

== system PubIfDecisionTOS_MDL/TOS_20201112/TOS_2012080320/TOS/ACC/TOS_ACCCurrentLane/ACC_CurrentLane_Target/TOS_ACC_P0/ACC_P0_Targe/ACC_P0_Targe/TOS_ACC_TargetMovingDirConfirm/TOS_ACC_TargetMovingDirConfirm_V2011170316(备份)/Subsystem ==
  ObjMovState : Inport
  ACC_Target_ID_K1 : Inport  Port=2
  ACC_Target_ID_K2 : Inport  Port=3
  ACC_Target_MovState_K1 : Inport  Port=4
  ACC_Target_MovState_K2 : Inport  Port=5
  ObjectID : Inport  Port=6
  TOS_ObjMovStateCfmFlow : Stateflow chart  TreatAsAtomicUnit=on
  TOS_ObjMovStateCfm : Outport
  wires:
  ObjectID/1 -> TOS_ObjMovStateCfmFlow/6(ObjectID)
  ObjMovState/1 -> TOS_ObjMovStateCfmFlow/5(ObjMovState)
  ACC_Target_MovState_K2/1 -> TOS_ObjMovStateCfmFlow/4(Target_MovState_K2)
  ACC_Target_MovState_K1/1 -> TOS_ObjMovStateCfmFlow/3(Target_MovState_K1)
  ACC_Target_ID_K2/1 -> TOS_ObjMovStateCfmFlow/2(Target_ID_K2)
  ACC_Target_ID_K1/1 -> TOS_ObjMovStateCfmFlow/1(Target_ID_K1)
  TOS_ObjMovStateCfmFlow/1(TOS_ObjMovStateCfm) -> TOS_ObjMovStateCfm/1

== system PubIfDecisionTOS_MDL/TOS_20201112/TOS_2012080320/TOS/ACC/TOS_ACCCurrentLane/ACC_CurrentLane_Target/TOS_ACC_P0/ACC_P0_Targe/ACC_P0_Targe/TOS_ACC_TargetMovingDirConfirm/TOS_ACC_TargetMovingDirConfirm_V2011170316(备份)/TOS_ACCMovingDirAborDly ==
  ACC_TargetP0_ID_K1 : Inport
  ObjectID : Inport  Port=2
  TOS_ACCMovingDir : Inport  Port=3
  If : If  IfExpression=u1
  If Action Subsystem : Subsystem  TreatAsAtomicUnit=on
  If Action Subsystem1 : Subsystem  TreatAsAtomicUnit=on
  Merge : Merge
  Subsystem : Subsystem
  TOS_ACC_TrgMovDirFlag_6_ObserVale : Outport
  TOS_ACC_TrgMovDir : Outport  Port=2
  wires:
  Merge/1 -> TOS_ACC_TrgMovDir/1
  If Action Subsystem/1(TOS_ACCMovingDirFilt) -> Merge/2
  If Action Subsystem1/1(TOS_ACCMovingDirFilt) -> Merge/1
  Subsystem/1(ACC_SameTargetP0) -> If/1, TOS_ACC_TrgMovDirFlag_6_ObserVale/1
  ObjectID/1 -> Subsystem/2(ObjectID)
  ACC_TargetP0_ID_K1/1 -> Subsystem/1(ACC_TargetP0_ID_K1)
  If/2 -> If Action Subsystem/Action
  TOS_ACCMovingDir/1 -> If Action Subsystem/1(TOS_ACCMovingDir), If Action Subsystem1/1(TOS_ACCMovingDir)
  If/1 -> If Action Subsystem1/Action

== system PubIfDecisionTOS_MDL/TOS_20201112/TOS_2012080320/TOS/ACC/TOS_ACCCurrentLane/ACC_CurrentLane_Target/TOS_ACC_P1/ACC_P1_Targe/ACC_P1_Targe/TOS_ACC_FusionTypeConfirm/TOS_ACCFusionTypeAborDly/If Action Subsystem ==
  TOS_ACCFusionType : Inport
  Action Port : ActionPort  ActionPortLabel=else
  TOS_ACCFusionTypeFilt : Outport
  wires:
  TOS_ACCFusionType/1 -> TOS_ACCFusionTypeFilt/1

== system PubIfDecisionTOS_MDL/TOS_20201112/TOS_2012080320/TOS/ACC/TOS_ACCCurrentLane/ACC_CurrentLane_Target/TOS_ACC_P1/ACC_P1_Targe/ACC_P1_Targe/TOS_ACC_FusionTypeConfirm/TOS_ACCFusionTypeAborDly/If Action Subsystem1 ==
  TOS_ACCFusionType : Inport
  Action Port : ActionPort  ActionPortLabel=if(u1)
  Constant : Constant  Value=0.15
  Constant4 : Constant  Value=0.05
  StateDelayAbortion : TOS_LIB/StateDelayAbortion  SystemSampleTime=-1  VariantActivationTime=update diagram  Latency=0  AutoFrameSizeCalculation=off
  TOS_ACCFusionTypeFilt : Outport
  wires:
  StateDelayAbortion/1 -> TOS_ACCFusionTypeFilt/1
  Constant/1 -> StateDelayAbortion/2
  Constant4/1 -> StateDelayAbortion/3
  TOS_ACCFusionType/1 -> StateDelayAbortion/1

== system PubIfDecisionTOS_MDL/TOS_20201112/TOS_2012080320/TOS/ACC/TOS_ACCCurrentLane/ACC_CurrentLane_Target/TOS_ACC_P1/ACC_P1_Targe/ACC_P1_Targe/TOS_ACC_ObjTypeConfirm/TOS_ACCObjTypeAborDly/If Action Subsystem ==
  TOS_ACCFusionType : Inport
  Action Port : ActionPort  ActionPortLabel=else
  TOS_ACCFusionTypeFilt : Outport
  wires:
  TOS_ACCFusionType/1 -> TOS_ACCFusionTypeFilt/1

== system PubIfDecisionTOS_MDL/TOS_20201112/TOS_2012080320/TOS/ACC/TOS_ACCCurrentLane/ACC_CurrentLane_Target/TOS_ACC_P1/ACC_P1_Targe/ACC_P1_Targe/TOS_ACC_ObjTypeConfirm/TOS_ACCObjTypeAborDly/If Action Subsystem1 ==
  TOS_ACCFusionType : Inport
  Action Port : ActionPort  ActionPortLabel=if(u1)
  Constant : Constant  Value=0.15
  Constant4 : Constant  Value=0.05
  StateDelayAbortion : TOS_LIB/StateDelayAbortion  SystemSampleTime=-1  VariantActivationTime=update diagram  Latency=0  AutoFrameSizeCalculation=off
  TOS_ACCFusionTypeFilt : Outport
  wires:
  StateDelayAbortion/1 -> TOS_ACCFusionTypeFilt/1
  Constant/1 -> StateDelayAbortion/2
  Constant4/1 -> StateDelayAbortion/3
  TOS_ACCFusionType/1 -> StateDelayAbortion/1

== system PubIfDecisionTOS_MDL/TOS_20201112/TOS_2012080320/TOS/ACC/TOS_ACCCurrentLane/ACC_CurrentLane_Target/TOS_ACC_P1/ACC_P1_Targe/ACC_P1_Targe/TOS_ACC_ObstacleProbConfirm/TOS_ACCObstacleProbAborDly/If Action Subsystem ==
  TOS_ACCFusionType : Inport
  Action Port : ActionPort  ActionPortLabel=else
  TOS_ACCFusionTypeFilt : Outport
  wires:
  TOS_ACCFusionType/1 -> TOS_ACCFusionTypeFilt/1

== system PubIfDecisionTOS_MDL/TOS_20201112/TOS_2012080320/TOS/ACC/TOS_ACCCurrentLane/ACC_CurrentLane_Target/TOS_ACC_P1/ACC_P1_Targe/ACC_P1_Targe/TOS_ACC_ObstacleProbConfirm/TOS_ACCObstacleProbAborDly/If Action Subsystem1 ==
  TOS_ACCFusionType : Inport
  Action Port : ActionPort  ActionPortLabel=if(u1)
  Constant : Constant  Value=0.15
  Constant4 : Constant  Value=0.05
  StateDelayAbortion : TOS_LIB/StateDelayAbortion  SystemSampleTime=-1  VariantActivationTime=update diagram  Latency=0  AutoFrameSizeCalculation=off
  TOS_ACCFusionTypeFilt : Outport
  wires:
  StateDelayAbortion/1 -> TOS_ACCFusionTypeFilt/1
  Constant/1 -> StateDelayAbortion/2
  Constant4/1 -> StateDelayAbortion/3
  TOS_ACCFusionType/1 -> StateDelayAbortion/1

== system PubIfDecisionTOS_MDL/TOS_20201112/TOS_2012080320/TOS/ACC/TOS_ACCCurrentLane/ACC_CurrentLane_Target/TOS_ACC_P1/ACC_P1_Targe/ACC_P1_Targe/TOS_ACC_ObstacleProbConfirm/TOS_ACCObstacleProbAborDly/Subsystem ==
  ACC_TargetP0_ID_K1 : Inport
  ObjectID : Inport  Port=2
  Relational Operator : RelationalOperator  Operator===  OutDataTypeStr=boolean  RndMeth=Simplest
  ACC_SameTargetP0 : Outport
  wires:
  ObjectID/1 -> Relational Operator/2
  Relational Operator/1 -> ACC_SameTargetP0/1
  ACC_TargetP0_ID_K1/1 -> Relational Operator/1

== system PubIfDecisionTOS_MDL/TOS_20201112/TOS_2012080320/TOS/ACC/TOS_ACCCurrentLane/ACC_CurrentLane_Target/TOS_ACC_P1/ACC_P1_Targe/ACC_P1_Targe/TOS_ACC_TargetMovingDirConfirm/TOS_ACCMovingDirAborDly/If Action Subsystem ==
  TOS_ACCMovingDir : Inport
  Action Port : ActionPort  ActionPortLabel=else
  TOS_ACCMovingDirFilt : Outport
  wires:
  TOS_ACCMovingDir/1 -> TOS_ACCMovingDirFilt/1

== system PubIfDecisionTOS_MDL/TOS_20201112/TOS_2012080320/TOS/ACC/TOS_ACCCurrentLane/ACC_CurrentLane_Target/TOS_ACC_P1/ACC_P1_Targe/ACC_P1_Targe/TOS_ACC_TargetMovingDirConfirm/TOS_ACCMovingDirAborDly/If Action Subsystem1 ==
  TOS_ACCMovingDir : Inport
  Action Port : ActionPort  ActionPortLabel=if(u1)
  Constant : Constant  Value=0.15
  Constant4 : Constant  Value=0.05
  StateDelayAbortion : TOS_LIB/StateDelayAbortion  SystemSampleTime=-1  VariantActivationTime=update diagram  Latency=0  AutoFrameSizeCalculation=off
  TOS_ACCMovingDirFilt : Outport
  wires:
  StateDelayAbortion/1 -> TOS_ACCMovingDirFilt/1
  Constant/1 -> StateDelayAbortion/2
  Constant4/1 -> StateDelayAbortion/3
  TOS_ACCMovingDir/1 -> StateDelayAbortion/1

== system PubIfDecisionTOS_MDL/TOS_20201112/TOS_2012080320/TOS/ACC/TOS_ACCCurrentLane/ACC_CurrentLane_Target/TOS_ACC_P1/ACC_P1_Targe/ACC_P1_Targe/TOS_ACC_TargetMovingDirConfirm/TOS_ACCMovingDirAborDly/Subsystem ==
  ACC_TargetP0_ID_K1 : Inport
  ObjectID : Inport  Port=2
  Relational Operator : RelationalOperator  Operator===  OutDataTypeStr=boolean  RndMeth=Simplest
  ACC_SameTargetP0 : Outport
  wires:
  ObjectID/1 -> Relational Operator/2
  Relational Operator/1 -> ACC_SameTargetP0/1
  ACC_TargetP0_ID_K1/1 -> Relational Operator/1

== system PubIfDecisionTOS_MDL/TOS_20201112/TOS_2012080320/TOS/ACC/TOS_ACCLeftLane/ACC_LeftLane_Target/TOS_ACC_P2/ACC_P2_Targe/ACC_P2_Targe/TOS_ACC_FusionTypeConfirm/TOS_ACCFusionTypeAborDly/If Action Subsystem ==
  TOS_ACCFusionType : Inport
  Action Port : ActionPort  ActionPortLabel=else
  TOS_ACCFusionTypeFilt : Outport
  wires:
  TOS_ACCFusionType/1 -> TOS_ACCFusionTypeFilt/1

== system PubIfDecisionTOS_MDL/TOS_20201112/TOS_2012080320/TOS/ACC/TOS_ACCLeftLane/ACC_LeftLane_Target/TOS_ACC_P2/ACC_P2_Targe/ACC_P2_Targe/TOS_ACC_FusionTypeConfirm/TOS_ACCFusionTypeAborDly/If Action Subsystem1 ==
  TOS_ACCFusionType : Inport
  Action Port : ActionPort  ActionPortLabel=if(u1)
  Constant : Constant  Value=0.15
  Constant4 : Constant  Value=0.05
  StateDelayAbortion : TOS_LIB/StateDelayAbortion  SystemSampleTime=-1  VariantActivationTime=update diagram  Latency=0  AutoFrameSizeCalculation=off
  TOS_ACCFusionTypeFilt : Outport
  wires:
  StateDelayAbortion/1 -> TOS_ACCFusionTypeFilt/1
  Constant/1 -> StateDelayAbortion/2
  Constant4/1 -> StateDelayAbortion/3
  TOS_ACCFusionType/1 -> StateDelayAbortion/1

== system PubIfDecisionTOS_MDL/TOS_20201112/TOS_2012080320/TOS/ACC/TOS_ACCLeftLane/ACC_LeftLane_Target/TOS_ACC_P2/ACC_P2_Targe/ACC_P2_Targe/TOS_ACC_ObjTypeConfirm/Subsystem1/Subsystem ==
  ObjMovState : Inport
  ACC_Target_ID_K1 : Inport  Port=2
  ACC_Target_ID_K2 : Inport  Port=3
  ACC_Target_MovState_K1 : Inport  Port=4
  ACC_Target_MovState_K2 : Inport  Port=5
  ObjectID : Inport  Port=6
  TOS_ObjMovStateCfmFlow1 : Stateflow chart  TreatAsAtomicUnit=on
  TOS_ObjMovStateCfm : Outport
  wires:
  ObjectID/1 -> TOS_ObjMovStateCfmFlow1/6(ObjectID)
  ObjMovState/1 -> TOS_ObjMovStateCfmFlow1/5(ObjMovState)
  ACC_Target_MovState_K2/1 -> TOS_ObjMovStateCfmFlow1/4(ACC_TargetP0_MovState_K2)
  ACC_Target_MovState_K1/1 -> TOS_ObjMovStateCfmFlow1/3(ACC_TargetP0_MovState_K1)
  ACC_Target_ID_K2/1 -> TOS_ObjMovStateCfmFlow1/2(ACC_TargetP0_ID_K2)
  ACC_Target_ID_K1/1 -> TOS_ObjMovStateCfmFlow1/1(ACC_TargetP0_ID_K1)
  TOS_ObjMovStateCfmFlow1/1(TOS_ObjMovStateCfm) -> TOS_ObjMovStateCfm/1

== system PubIfDecisionTOS_MDL/TOS_20201112/TOS_2012080320/TOS/ACC/TOS_ACCLeftLane/ACC_LeftLane_Target/TOS_ACC_P2/ACC_P2_Targe/ACC_P2_Targe/TOS_ACC_ObjTypeConfirm/TOS_ACCObjTypeAborDly/If Action Subsystem ==
  TOS_ACCFusionType : Inport
  Action Port : ActionPort  ActionPortLabel=else
  TOS_ACCFusionTypeFilt : Outport
  wires:
  TOS_ACCFusionType/1 -> TOS_ACCFusionTypeFilt/1

== system PubIfDecisionTOS_MDL/TOS_20201112/TOS_2012080320/TOS/ACC/TOS_ACCLeftLane/ACC_LeftLane_Target/TOS_ACC_P2/ACC_P2_Targe/ACC_P2_Targe/TOS_ACC_ObjTypeConfirm/TOS_ACCObjTypeAborDly/If Action Subsystem1 ==
  TOS_ACCFusionType : Inport
  Action Port : ActionPort  ActionPortLabel=if(u1)
  Constant : Constant  Value=0.15
  Constant4 : Constant  Value=0.05
  StateDelayAbortion : TOS_LIB/StateDelayAbortion  SystemSampleTime=-1  VariantActivationTime=update diagram  Latency=0  AutoFrameSizeCalculation=off
  TOS_ACCFusionTypeFilt : Outport
  wires:
  StateDelayAbortion/1 -> TOS_ACCFusionTypeFilt/1
  Constant/1 -> StateDelayAbortion/2
  Constant4/1 -> StateDelayAbortion/3
  TOS_ACCFusionType/1 -> StateDelayAbortion/1

== system PubIfDecisionTOS_MDL/TOS_20201112/TOS_2012080320/TOS/ACC/TOS_ACCLeftLane/ACC_LeftLane_Target/TOS_ACC_P2/ACC_P2_Targe/ACC_P2_Targe/TOS_ACC_ObstacleProbConfirm/TOS_ACCObstacleProbAborDly/If Action Subsystem ==
  TOS_ACCFusionType : Inport
  Action Port : ActionPort  ActionPortLabel=else
  TOS_ACCFusionTypeFilt : Outport
  wires:
  TOS_ACCFusionType/1 -> TOS_ACCFusionTypeFilt/1

== system PubIfDecisionTOS_MDL/TOS_20201112/TOS_2012080320/TOS/ACC/TOS_ACCLeftLane/ACC_LeftLane_Target/TOS_ACC_P2/ACC_P2_Targe/ACC_P2_Targe/TOS_ACC_ObstacleProbConfirm/TOS_ACCObstacleProbAborDly/If Action Subsystem1 ==
  TOS_ACCFusionType : Inport
  Action Port : ActionPort  ActionPortLabel=if(u1)
  Constant : Constant  Value=0.15
  Constant4 : Constant  Value=0.05
  StateDelayAbortion : TOS_LIB/StateDelayAbortion  SystemSampleTime=-1  VariantActivationTime=update diagram  Latency=0  AutoFrameSizeCalculation=off
  TOS_ACCFusionTypeFilt : Outport
  wires:
  StateDelayAbortion/1 -> TOS_ACCFusionTypeFilt/1
  Constant/1 -> StateDelayAbortion/2
  Constant4/1 -> StateDelayAbortion/3
  TOS_ACCFusionType/1 -> StateDelayAbortion/1

== system PubIfDecisionTOS_MDL/TOS_20201112/TOS_2012080320/TOS/ACC/TOS_ACCLeftLane/ACC_LeftLane_Target/TOS_ACC_P2/ACC_P2_Targe/ACC_P2_Targe/TOS_ACC_ObstacleProbConfirm/TOS_ACCObstacleProbAborDly/Subsystem ==
  ACC_TargetP0_ID_K1 : Inport
  ObjectID : Inport  Port=2
  Relational Operator : RelationalOperator  Operator===  OutDataTypeStr=boolean  RndMeth=Simplest
  ACC_SameTargetP0 : Outport
  wires:
  ObjectID/1 -> Relational Operator/2
  Relational Operator/1 -> ACC_SameTargetP0/1
  ACC_TargetP0_ID_K1/1 -> Relational Operator/1

== system PubIfDecisionTOS_MDL/TOS_20201112/TOS_2012080320/TOS/ACC/TOS_ACCLeftLane/ACC_LeftLane_Target/TOS_ACC_P2/ACC_P2_Targe/ACC_P2_Targe/TOS_ACC_TargetMovingDirConfirm/TOS_ACCMovingDirAborDly/If Action Subsystem ==
  TOS_ACCMovingDir : Inport
  Action Port : ActionPort  ActionPortLabel=else
  TOS_ACCMovingDirFilt : Outport
  wires:
  TOS_ACCMovingDir/1 -> TOS_ACCMovingDirFilt/1

== system PubIfDecisionTOS_MDL/TOS_20201112/TOS_2012080320/TOS/ACC/TOS_ACCLeftLane/ACC_LeftLane_Target/TOS_ACC_P2/ACC_P2_Targe/ACC_P2_Targe/TOS_ACC_TargetMovingDirConfirm/TOS_ACCMovingDirAborDly/If Action Subsystem1 ==
  TOS_ACCMovingDir : Inport
  Action Port : ActionPort  ActionPortLabel=if(u1)
  Constant : Constant  Value=0.15
  Constant4 : Constant  Value=0.05
  StateDelayAbortion : TOS_LIB/StateDelayAbortion  SystemSampleTime=-1  VariantActivationTime=update diagram  Latency=0  AutoFrameSizeCalculation=off
  TOS_ACCMovingDirFilt : Outport
  wires:
  StateDelayAbortion/1 -> TOS_ACCMovingDirFilt/1
  Constant/1 -> StateDelayAbortion/2
  Constant4/1 -> StateDelayAbortion/3
  TOS_ACCMovingDir/1 -> StateDelayAbortion/1

== system PubIfDecisionTOS_MDL/TOS_20201112/TOS_2012080320/TOS/ACC/TOS_ACCLeftLane/ACC_LeftLane_Target/TOS_ACC_P2/ACC_P2_Targe/ACC_P2_Targe/TOS_ACC_TargetMovingDirConfirm/TOS_ACCMovingDirAborDly/Subsystem ==
  ACC_TargetP0_ID_K1 : Inport
  ObjectID : Inport  Port=2
  Relational Operator : RelationalOperator  Operator===  OutDataTypeStr=boolean  RndMeth=Simplest
  ACC_SameTargetP0 : Outport
  wires:
  ObjectID/1 -> Relational Operator/2
  Relational Operator/1 -> ACC_SameTargetP0/1
  ACC_TargetP0_ID_K1/1 -> Relational Operator/1

== system PubIfDecisionTOS_MDL/TOS_20201112/TOS_2012080320/TOS/ACC/TOS_ACCLeftLane/ACC_LeftLane_Target/TOS_ACC_P4/ACC_P4_Targe/ACC_P4_Targe/TOS_ACC_FusionTypeConfirm/TOS_ACCFusionTypeAborDly/If Action Subsystem ==
  TOS_ACCFusionType : Inport
  Action Port : ActionPort  ActionPortLabel=else
  TOS_ACCFusionTypeFilt : Outport
  wires:
  TOS_ACCFusionType/1 -> TOS_ACCFusionTypeFilt/1

== system PubIfDecisionTOS_MDL/TOS_20201112/TOS_2012080320/TOS/ACC/TOS_ACCLeftLane/ACC_LeftLane_Target/TOS_ACC_P4/ACC_P4_Targe/ACC_P4_Targe/TOS_ACC_FusionTypeConfirm/TOS_ACCFusionTypeAborDly/If Action Subsystem1 ==
  TOS_ACCFusionType : Inport
  Action Port : ActionPort  ActionPortLabel=if(u1)
  Constant : Constant  Value=0.15
  Constant4 : Constant  Value=0.05
  StateDelayAbortion : TOS_LIB/StateDelayAbortion  SystemSampleTime=-1  VariantActivationTime=update diagram  Latency=0  AutoFrameSizeCalculation=off
  TOS_ACCFusionTypeFilt : Outport
  wires:
  TOS_ACCFusionType/1 -> StateDelayAbortion/1
  Constant4/1 -> StateDelayAbortion/3
  Constant/1 -> StateDelayAbortion/2
  StateDelayAbortion/1 -> TOS_ACCFusionTypeFilt/1
